simulink model "Twin_SL_RC"  (R2026a)
settings: Solver=ode4  StartTime=0  StopTime=4.1e-6  FixedStep=9.9999999999999998e-13
settings Model: Creator=35609  LastModifiedBy=35609

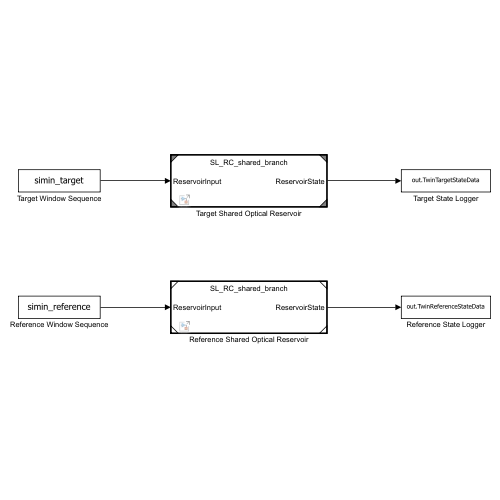
[thumbnail: Simulink's stored preview of the top-level diagram]
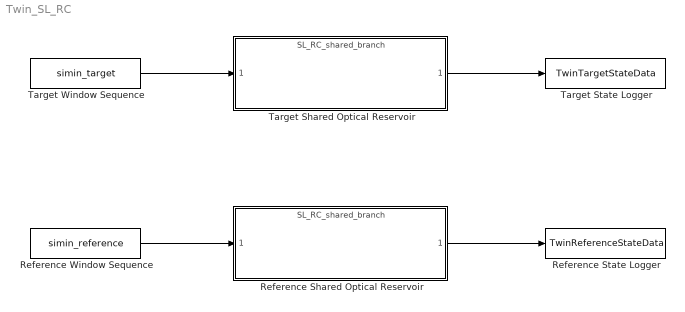
== system Twin_SL_RC ==
  Reference Shared Optical Reservoir : ModelReference  ModelNameDialog=SL_RC_shared_branch  SimulationMode=Normal  ModelReferenceVersion=21.8
  Reference State Logger : ToWorkspace  VariableName=TwinReferenceStateData  SaveFormat=Timeseries  SampleTime=3.9999999999999998e-11
  Reference Window Sequence : FromWorkspace  VariableName=simin_reference
  Target Shared Optical Reservoir : ModelReference  ModelNameDialog=SL_RC_shared_branch  SimulationMode=Normal  ModelReferenceVersion=21.8
  Target State Logger : ToWorkspace  VariableName=TwinTargetStateData  SaveFormat=Timeseries  SampleTime=3.9999999999999998e-11
  Target Window Sequence : FromWorkspace  VariableName=simin_target
  wires:
  Target Window Sequence/1 -> Target Shared Optical Reservoir/1
  Reference Window Sequence/1 -> Reference Shared Optical Reservoir/1
  Target Shared Optical Reservoir/1 -> Target State Logger/1
  Reference Shared Optical Reservoir/1 -> Reference State Logger/1
